simulink model "uz_FOC"  (R2021a)
settings: Solver=FixedStepDiscrete  StartTime=0.0  StopTime=50.0  FixedStep=0.00001  RelTol=1e-3  EnableMultiTasking=on
values from neighbouring files (symbols this model uses):
  d_d_TMS = 0.005    [uz_FOC_init.m]
  d_f_c = 100000    [uz_FOC_init.m]
  d_i_max = 15    [uz_FOC_init.m]
  d_i_min = -d_i_max    (= -15)    [uz_FOC_init.m]
  d_J_Coupling_M_E = 2e-6    (= 2e-06)    [uz_FOC_init.m]
  d_J_Coupling_M_Ms = 2e-20    [uz_FOC_init.m]
  d_J_Ms_L = d_J_Ms_M    (= 1.26363648e-05)    [uz_FOC_init.m]
  d_J_Ms_M = 0.5*0.5*((0.5*d_d_Ms)^4)*3.14*d_l_Ms*d_rho_Ms    (= 1.26363648e-05)    [uz_FOC_init.m]
  d_Ki_id = d_Kp_id/d_Tn_id    (= 125)    [uz_FOC_init.m]
  d_Ki_iq = d_Kp_iq/d_Tn_iq    (= 125)    [uz_FOC_init.m]
  d_Ki_n = d_Kp_n/d_Tn_n    (= 0.003888)    [uz_FOC_init.m]
  d_Kp_id = d_L_d / (4*20/d_f_c)    (= 0.25)    [uz_FOC_init.m]
  d_Kp_iq = d_L_q / (4*20/d_f_c)    (= 0.375)    [uz_FOC_init.m]
  d_Kp_n = 0.00864*0.045    (= 0.0003888)    [uz_FOC_init.m]
  d_L_d = 0.0002    [uz_FOC_init.m]
  d_L_q = 0.0003    [uz_FOC_init.m]
  d_p = 4    [uz_FOC_init.m]
  d_psi_pm = 0.0075    [uz_FOC_init.m]
  d_R_ph = d_R_ph_ph/2    (= 0.1)    [uz_FOC_init.m]
  d_y_max = 10    [uz_FOC_init.m]
  d_y_min = -d_y_max    (= -10)    [uz_FOC_init.m]
undefined symbols (not defined in the file or in its folder): i_d, i_q, para, u_d, u_q
libraries: fl_lib x44, nesl_utility x27, ee_lib x21, simulink x8, spsabctodq0Lib x2, spsTriangleGeneratorLib x1, eeTransforms x1
(part 3 of 3)

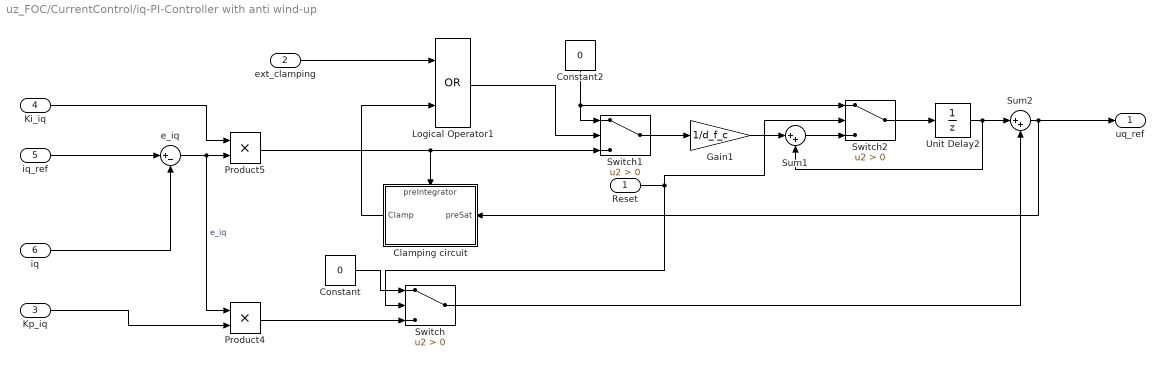
== system uz_FOC/CurrentControl/iq-PI-Controller with anti wind-up ==
  Reset : Inport
  ext_clamping : Inport  Port=2
  Kp_iq : Inport  Port=3
  Ki_iq : Inport  Port=4
  iq_ref : Inport  Port=5
  iq : Inport  Port=6
  Clamping circuit : Subsystem
      settings: PortSchema="{\"entries\":[{\"content\":{\"sides\":[{\"content\":{\"connectorIds\":[\"In1\"]},\"type\":\"ConnectorPlacement.EquallySpacedRectSide\",\"uuid\":\"9b5eb3d3-336d-4b55-a615-0420b1cf4a48\"},{\"content\":{\"connectorIds\":[\"Out1\"],\"side\":\"RIGHT\"},\"type\":\"ConnectorPlacement.EquallySpacedRectSide\",\"uuid\":\"a73559ab-79dd-4c84-b45a-6a43ba4812e9\"},{\"content\":{\"connectorIds\":[\"In2\"],\"side\":\"TOP\"},\"type\":\"ConnectorPlacement.EquallySpacedRectSide\",\"uuid\":\"82c30f31-c271-4a2b-89be-8686aa9e20f3\"}]},\"type\":\"ConnectorPlacement.EquallySpacedConnector\",\"uuid\":\"376d2fe4-39b3-495b-8d80-8756076e2730\"}],\"packageUris\":[\"http://schema.mathworks.com/mf0/Connector/R2020b\"],\"version\":\"1.0\"}"
  Constant : Constant  Value=0  SampleTime=1/d_f_c
  Constant2 : Constant  Value=0  SampleTime=1/d_f_c
  Gain1 : Gain  Gain=1/d_f_c
  Logical Operator1 : Logic  Operator=OR  AllPortsSameDT=off  OutDataTypeStr=boolean
  Product4 : Product
  Product5 : Product
  Sum1 : Sum  Inputs=|++  OutDataTypeStr=single
  Sum2 : Sum  Inputs=|++  OutDataTypeStr=single
  Switch : Switch  Criteria=u2 > Threshold
  Switch1 : Switch  Criteria=u2 > Threshold
  Switch2 : Switch  Criteria=u2 > Threshold
  Unit Delay2 : UnitDelay  SampleTime=-1  HasFrameUpgradeWarning=on
  e_iq : Sum  Inputs=|+-
  uq_ref : Outport
  wires:
  ext_clamping/1 -> Logical Operator1/1
  Kp_iq/1 -> Product4/2
  Ki_iq/1 -> Product5/1
  iq_ref/1 -> e_iq/1
  iq/1 -> e_iq/2
  e_iq/1 -> Product5/2, Product4/1  "e_iq"
  Unit Delay2/1 -> Sum2/1, Sum1/2
  Clamping circuit/1(Clamp) -> Logical Operator1/2
  Sum2/1 -> uq_ref/1, Clamping circuit/1(preSat)
  Switch/1 -> Sum2/2
  Constant/1 -> Switch/1
  Product4/1 -> Switch/3
  Switch2/1 -> Unit Delay2/1
  Gain1/1 -> Sum1/1
  Constant2/1 -> Switch2/1, Switch1/1
  Sum1/1 -> Switch2/3
  Product5/1 -> Switch1/3, Clamping circuit/2(preIntegrator)
  Switch1/1 -> Gain1/1
  Reset/1 -> Switch2/2, Switch/2
  Logical Operator1/1 -> Switch1/2

== system uz_FOC/CurrentControl/linear decouppling ==
  i_q : Inport
  i_d : Inport  Port=2
  omega_el : Inport  Port=3
  Gain : Gain  Gain=-d_L_q
  Gain4 : Gain  Gain=d_L_d
  Product : Product  SaturateOnIntegerOverflow=on
  Product1 : Product  SaturateOnIntegerOverflow=on
  Sum : Sum  Inputs=|++
  d_psi_pm : Constant  Value=d_psi_pm  OutDataTypeStr=Inherit: Inherit via back propagation  SampleTime=1/d_f_c
  u_d_vor : Outport  VectorParamsAs1DForOutWhenUnconnected=off
  u_q_vor : Outport  Port=2  VectorParamsAs1DForOutWhenUnconnected=off
  wires:
  i_q/1 -> Product/1
  Product1/1 -> u_q_vor/1
  Gain/1 -> Product/2
  Sum/1 -> Product1/1
  Product/1 -> u_d_vor/1
  omega_el/1 -> Gain/1, Product1/2
  Gain4/1 -> Sum/1
  d_psi_pm/1 -> Sum/2
  i_d/1 -> Gain4/1

== system uz_FOC/CurrentControl/nonlinear decouppling ==
  i_q : Inport
  i_d : Inport  Port=2
  omega_el : Inport  Port=3
  Gain12 : Gain  Gain=-1
  Product1 : Product
  Product8 : Product
  psi_d(u1=id,u2=iq) : Lookup_n-D  BreakpointsForDimension1=para.id_LUT  BreakpointsForDimension2=para.iq_LUT  Table=para.psi_q  InterpMethod=Cubic spline  ExtrapMethod=Clip  InternalRulePriority=Speed  RndMeth=Simplest  InputSameDT=on
      settings: InputPortMap=u0,u1
  psi_q(u1=id,u2=iq) : Lookup_n-D  BreakpointsForDimension1=para.id_LUT  BreakpointsForDimension2=para.iq_LUT  Table=para.psi_q  InterpMethod=Cubic spline  ExtrapMethod=Clip  InternalRulePriority=Speed  RndMeth=Simplest  InputSameDT=on
      settings: InputPortMap=u0,u1
  ud_vor : Outport  VectorParamsAs1DForOutWhenUnconnected=off
  uq_vor : Outport  Port=2  VectorParamsAs1DForOutWhenUnconnected=off
  wires:
  i_q/1 -> psi_q(u1=id,u2=iq)/2, psi_d(u1=id,u2=iq)/2
  i_d/1 -> psi_d(u1=id,u2=iq)/1, psi_q(u1=id,u2=iq)/1
  Product1/1 -> uq_vor/1
  Gain12/1 -> ud_vor/1
  Product8/1 -> Gain12/1
  psi_d(u1=id,u2=iq)/1 -> Product1/2
  omega_el/1 -> Product8/1, Product1/1
  psi_q(u1=id,u2=iq)/1 -> Product8/2

== system uz_FOC/Hardware/Coupling Encoder ==
  note: 1) Add Subsystem or Model blocks as valid variant choices.
      | 2) You cannot connect blocks at this level. At simulation, connectivity is automatically
      | determined, based on the active variant and port name matching.
  Inertia : Subsystem  VariantControl=(default)
  Spring Damper System : Subsystem  VariantControl=TMS1
  Input : PMIOPort  Side=Left
  output : PMIOPort  Port=2  Side=Right

== system uz_FOC/Hardware/Measurement Shaft ==
  note: 1) Add Subsystem or Model blocks as valid variant choices.
      | 2) You cannot connect blocks at this level. At simulation, connectivity is automatically
      | determined, based on the active variant and port name matching.
  Spring Damper System : Subsystem  VariantControl=TMS1
  default : Subsystem  VariantControl=(default)
  Input : PMIOPort  Side=Left
  output : PMIOPort  Port=2  Side=Right

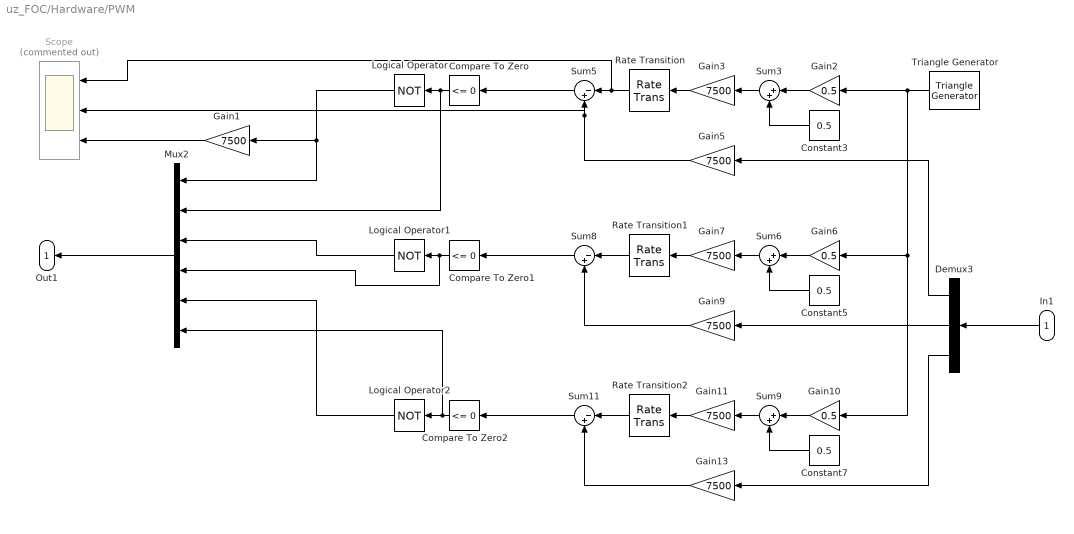
== system uz_FOC/Hardware/PWM ==
  In1 : Inport
  Compare To Zero : simulink/Logic and Bit Operations/Compare To Zero  relop=<=  OutDataTypeStr=boolean
  Compare To Zero1 : simulink/Logic and Bit Operations/Compare To Zero  relop=<=  OutDataTypeStr=boolean
  Compare To Zero2 : simulink/Logic and Bit Operations/Compare To Zero  relop=<=  OutDataTypeStr=boolean
  Constant3 : Constant  Value=0.5
  Constant5 : Constant  Value=0.5
  Constant7 : Constant  Value=0.5
  Demux3 : Demux  Outputs=3
  Gain{1,3,5,7,9,11,13} (7 alike) : Gain  Gain=7500  ParamDataTypeStr=single
  Gain10 : Gain  Gain=0.5
  Gain2 : Gain  Gain=0.5
  Gain6 : Gain  Gain=0.5
  Logical Operator : Logic  Operator=NOT  AllPortsSameDT=off  OutDataTypeStr=boolean
  Logical Operator1 : Logic  Operator=NOT  AllPortsSameDT=off  OutDataTypeStr=boolean
  Logical Operator2 : Logic  Operator=NOT  AllPortsSameDT=off  OutDataTypeStr=boolean
  Mux2 : Mux  Inputs=6
  Rate Transition : RateTransition  OutPortSampleTime=0.00001
  Rate Transition1 : RateTransition  OutPortSampleTime=0.00001
  Rate Transition2 : RateTransition  OutPortSampleTime=0.00001
  Scope : Scope  Commented=on  NumInputPorts=3
  Sum11 : Sum  Inputs=|-+
  Sum3 : Sum  Inputs=|++
  Sum5 : Sum  Inputs=|-+
  Sum6 : Sum  Inputs=|++
  Sum8 : Sum  Inputs=|-+
  Sum9 : Sum  Inputs=|++
  Triangle Generator : spsTriangleGeneratorLib/Triangle Generator  Freq=10000  Phase=0  Ts=0
  Out1 : Outport  VectorParamsAs1DForOutWhenUnconnected=off
  wires:
  Demux3/3 -> Gain13/1
  Logical Operator2/1 -> Mux2/5
  Logical Operator1/1 -> Mux2/3
  Mux2/1 -> Out1/1
  Compare To Zero2/1 -> Mux2/6, Logical Operator2/1
  Gain10/1 -> Sum9/1
  Sum8/1 -> Compare To Zero1/1
  Gain6/1 -> Sum6/1
  Sum9/1 -> Gain11/1
  Triangle Generator/1 -> Gain10/1, Gain6/1, Gain2/1
  Sum6/1 -> Gain7/1
  Demux3/2 -> Gain9/1
  Compare To Zero1/1 -> Mux2/4, Logical Operator1/1
  Constant5/1 -> Sum6/2
  Constant7/1 -> Sum9/2
  Sum11/1 -> Compare To Zero2/1
  Sum3/1 -> Gain3/1
  Constant3/1 -> Sum3/2
  Demux3/1 -> Gain5/1
  Sum5/1 -> Compare To Zero/1
  Gain2/1 -> Sum3/1
  In1/1 -> Demux3/1
  Gain3/1 -> Rate Transition/1
  Gain7/1 -> Rate Transition1/1
  Gain11/1 -> Rate Transition2/1
  Gain5/1 -> Scope/2, Sum5/2
  Gain9/1 -> Sum8/2
  Gain13/1 -> Sum11/2
  Rate Transition/1 -> Scope/1, Sum5/1
  Rate Transition1/1 -> Sum8/1
  Rate Transition2/1 -> Sum11/1
  Logical Operator/1 -> Gain1/1, Mux2/1
  Compare To Zero/1 -> Mux2/2, Logical Operator/1
  Gain1/1 -> Scope/3

== system uz_FOC/Hardware/Switch f. TMS ==
  note: 1) Add Subsystem or Model blocks as valid variant choices.
      | 2) You cannot connect blocks at this level. At simulation, connectivity is automatically
      | determined, based on the active variant and port name matching.
  closed : Subsystem  VariantControl=d_KupplZus==1
  open : Subsystem  VariantControl=d_KupplZus==0
  Input : PMIOPort  Side=Left
  output : PMIOPort  Port=2  Side=Right

== system uz_FOC/Hardware/coupling m. shaft ==
  note: 1) Add Subsystem or Model blocks as valid variant choices.
      | 2) You cannot connect blocks at this level. At simulation, connectivity is automatically
      | determined, based on the active variant and port name matching.
  Inertia : Subsystem  VariantControl=(default)
  Spring Damper System : Subsystem  VariantControl=TMS1
  Input : PMIOPort  Side=Left
  output : PMIOPort  Port=2  Side=Right

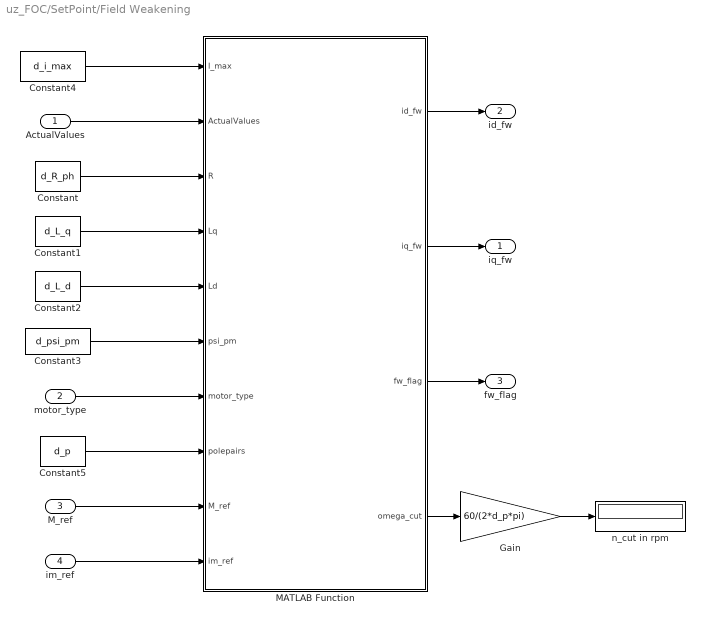
== system uz_FOC/SetPoint/Field Weakening ==
  ActualValues : Inport  OutDataTypeStr=single
  motor_type : Inport  Port=2  OutDataTypeStr=uint16
  M_ref : Inport  Port=3  OutDataTypeStr=single
  im_ref : Inport  Port=4  OutDataTypeStr=single
  Constant : Constant  Value=d_R_ph  OutDataTypeStr=single
  Constant1 : Constant  Value=d_L_q  OutDataTypeStr=single
  Constant2 : Constant  Value=d_L_d  OutDataTypeStr=single
  Constant3 : Constant  Value=d_psi_pm  OutDataTypeStr=single
  Constant4 : Constant  Value=d_i_max  OutDataTypeStr=single
  Constant5 : Constant  Value=d_p  OutDataTypeStr=single
  Gain : Gain  Gain=60/(2*d_p*pi)
  MATLAB Function : MATLAB Function  TreatAsAtomicUnit=on
  n_cut in rpm : Display
  iq_fw : Outport  OutDataTypeStr=single
  id_fw : Outport  Port=2  OutDataTypeStr=single
  fw_flag : Outport  Port=3  OutDataTypeStr=boolean
  wires:
  Constant4/1 -> MATLAB Function/1(I_max)
  ActualValues/1 -> MATLAB Function/2(ActualValues)
  Constant/1 -> MATLAB Function/3(R)
  Constant1/1 -> MATLAB Function/4(Lq)
  Constant2/1 -> MATLAB Function/5(Ld)
  Constant3/1 -> MATLAB Function/6(psi_pm)
  MATLAB Function/2(iq_fw) -> iq_fw/1
  MATLAB Function/1(id_fw) -> id_fw/1
  motor_type/1 -> MATLAB Function/7(motor_type)
  MATLAB Function/3(fw_flag) -> fw_flag/1
  M_ref/1 -> MATLAB Function/9(M_ref)
  im_ref/1 -> MATLAB Function/10(im_ref)
  Constant5/1 -> MATLAB Function/8(polepairs)
  MATLAB Function/4(omega_cut) -> Gain/1
  Gain/1 -> n_cut in rpm/1

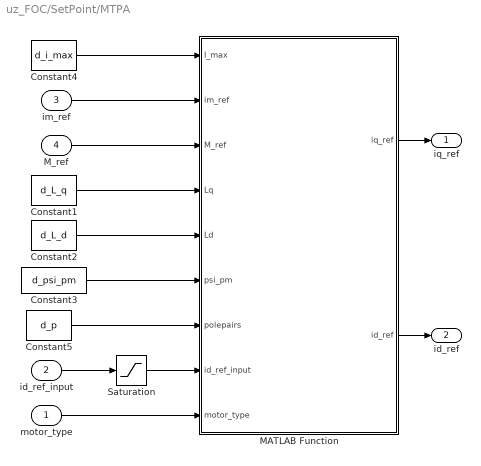
== system uz_FOC/SetPoint/MTPA ==
  motor_type : Inport  OutDataTypeStr=uint16
  id_ref_input : Inport  Port=2  OutDataTypeStr=single
  im_ref : Inport  Port=3  OutDataTypeStr=single
  M_ref : Inport  Port=4  OutDataTypeStr=single
  Constant1 : Constant  Value=d_L_q  OutDataTypeStr=single
  Constant2 : Constant  Value=d_L_d  OutDataTypeStr=single
  Constant3 : Constant  Value=d_psi_pm  OutDataTypeStr=single
  Constant4 : Constant  Value=d_i_max  OutDataTypeStr=single
  Constant5 : Constant  Value=d_p  OutDataTypeStr=single
  MATLAB Function : MATLAB Function  TreatAsAtomicUnit=on
  Saturation : Saturate  UpperLimit=d_i_max  LowerLimit=d_i_min
  iq_ref : Outport  OutDataTypeStr=single
  id_ref : Outport  Port=2  OutDataTypeStr=single
  wires:
  Constant4/1 -> MATLAB Function/1(I_max)
  Constant1/1 -> MATLAB Function/4(Lq)
  Constant2/1 -> MATLAB Function/5(Ld)
  Constant3/1 -> MATLAB Function/6(psi_pm)
  MATLAB Function/2(id_ref) -> id_ref/1
  MATLAB Function/1(iq_ref) -> iq_ref/1
  id_ref_input/1 -> Saturation/1
  Saturation/1 -> MATLAB Function/8(id_ref_input)
  im_ref/1 -> MATLAB Function/2(im_ref)
  motor_type/1 -> MATLAB Function/9(motor_type)
  Constant5/1 -> MATLAB Function/7(polepairs)
  M_ref/1 -> MATLAB Function/3(M_ref)

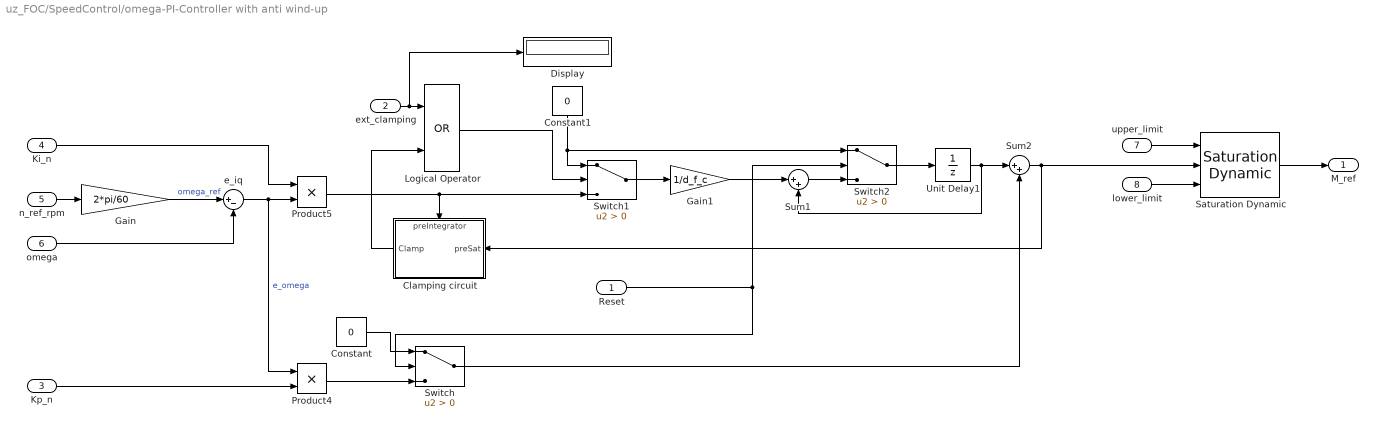
== system uz_FOC/SpeedControl/omega-PI-Controller with anti wind-up ==
  Reset : Inport
  ext_clamping : Inport  Port=2
  Kp_n : Inport  Port=3
  Ki_n : Inport  Port=4
  n_ref_rpm : Inport  Port=5
  omega : Inport  Port=6
  upper_limit : Inport  Port=7
  lower_limit : Inport  Port=8
  Clamping circuit : Subsystem
      settings: PortSchema="{\"entries\":[{\"content\":{\"sides\":[{\"content\":{\"connectorIds\":[\"In1\"]},\"type\":\"ConnectorPlacement.EquallySpacedRectSide\",\"uuid\":\"9b5eb3d3-336d-4b55-a615-0420b1cf4a48\"},{\"content\":{\"connectorIds\":[\"Out1\"],\"side\":\"RIGHT\"},\"type\":\"ConnectorPlacement.EquallySpacedRectSide\",\"uuid\":\"a73559ab-79dd-4c84-b45a-6a43ba4812e9\"},{\"content\":{\"connectorIds\":[\"In2\"],\"side\":\"TOP\"},\"type\":\"ConnectorPlacement.EquallySpacedRectSide\",\"uuid\":\"82c30f31-c271-4a2b-89be-8686aa9e20f3\"}]},\"type\":\"ConnectorPlacement.EquallySpacedConnector\",\"uuid\":\"376d2fe4-39b3-495b-8d80-8756076e2730\"}],\"packageUris\":[\"http://schema.mathworks.com/mf0/Connector/R2020b\"],\"version\":\"1.0\"}"
  Constant : Constant  Value=0  SampleTime=1/d_f_c
  Constant1 : Constant  Value=0  SampleTime=1/d_f_c
  Display : Display
  Gain : Gain  Gain=2*pi/60
  Gain1 : Gain  Gain=1/d_f_c
  Logical Operator : Logic  Operator=OR  AllPortsSameDT=off  OutDataTypeStr=boolean
  Product4 : Product
  Product5 : Product
  Saturation Dynamic : simulink/Discontinuities/Saturation Dynamic  OutMin=[]  OutMax=[]  OutDataTypeStr=Inherit: Same as second input  OutDataType=fixdt(1, 16)  OutScaling=2^-10  DoSatur=off
  Sum1 : Sum  Inputs=|++  OutDataTypeStr=single
  Sum2 : Sum  Inputs=|++  OutDataTypeStr=single
  Switch : Switch  Criteria=u2 > Threshold
  Switch1 : Switch  Criteria=u2 > Threshold
  Switch2 : Switch  Criteria=u2 > Threshold  OutDataTypeStr=single
  Unit Delay1 : UnitDelay  SampleTime=-1  HasFrameUpgradeWarning=on
  e_iq : Sum  Inputs=|+-  OutDataTypeStr=single
  M_ref : Outport
  wires:
  Kp_n/1 -> Product4/2
  Ki_n/1 -> Product5/1
  Gain/1 -> e_iq/1  "omega_ref"
  omega/1 -> e_iq/2
  e_iq/1 -> Product5/2, Product4/1  "e_omega"
  Switch/1 -> Sum2/2
  Unit Delay1/1 -> Sum2/1, Sum1/2
  Sum2/1 -> Clamping circuit/1(preSat), Saturation Dynamic/2
  ext_clamping/1 -> Display/1, Logical Operator/1
  Product5/1 -> Switch1/3, Clamping circuit/2(preIntegrator)
  Clamping circuit/1(Clamp) -> Logical Operator/2
  Constant/1 -> Switch/1
  Reset/1 -> Switch/2, Switch2/2
  Product4/1 -> Switch/3
  Constant1/1 -> Switch2/1, Switch1/1
  Logical Operator/1 -> Switch1/2
  n_ref_rpm/1 -> Gain/1
  Switch1/1 -> Gain1/1
  Gain1/1 -> Sum1/1
  Switch2/1 -> Unit Delay1/1
  Sum1/1 -> Switch2/3
  Saturation Dynamic/1 -> M_ref/1
  upper_limit/1 -> Saturation Dynamic/1
  lower_limit/1 -> Saturation Dynamic/3

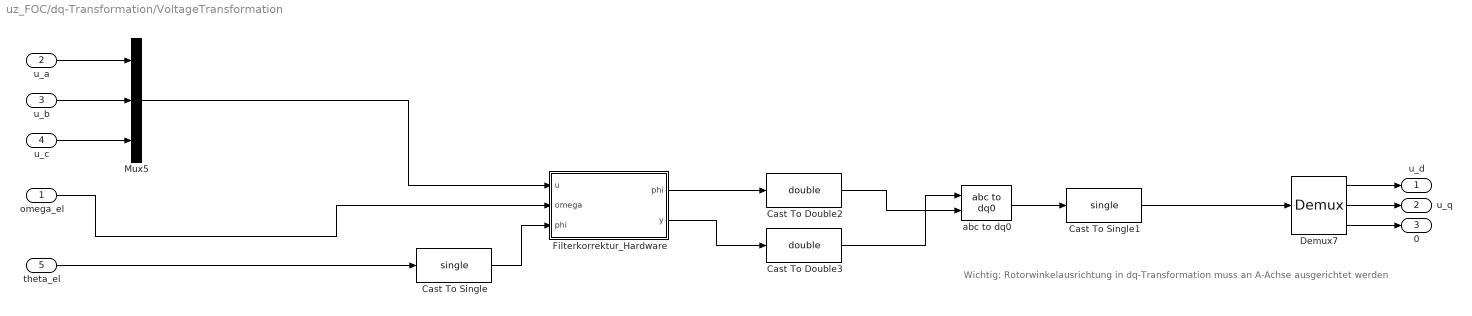
== system uz_FOC/dq-Transformation/VoltageTransformation ==
  note: Wichtig: Rotorwinkelausrichtung in dq-Transformation
      | muss an A-Achse ausgerichtet werden
  omega_el : Inport
  u_a : Inport  Port=2
  u_b : Inport  Port=3
  u_c : Inport  Port=4
  theta_el : Inport  Port=5
  Cast To Double2 : DataTypeConversion  OutDataTypeStr=double
  Cast To Double3 : DataTypeConversion  OutDataTypeStr=double
  Cast To Single : DataTypeConversion  OutDataTypeStr=single
  Cast To Single1 : DataTypeConversion  OutDataTypeStr=single
  Demux7 : Demux  Outputs=3
  Filterkorrektur_Hardware : MATLAB Function  TreatAsAtomicUnit=on
  Mux5 : Mux  Inputs=3
  abc to dq0 : spsabctodq0Lib/abc to dq0  Alignment=Aligned with phase A axis
  u_d : Outport  VectorParamsAs1DForOutWhenUnconnected=off
  u_q : Outport  Port=2  VectorParamsAs1DForOutWhenUnconnected=off
  0 : Outport  Port=3  VectorParamsAs1DForOutWhenUnconnected=off
  wires:
  Demux7/1 -> u_d/1
  Cast To Single/1 -> Filterkorrektur_Hardware/3("phi ")
  theta_el/1 -> Cast To Single/1
  Mux5/1 -> Filterkorrektur_Hardware/1(u)
  omega_el/1 -> Filterkorrektur_Hardware/2(omega)
  u_a/1 -> Mux5/1
  u_c/1 -> Mux5/3
  u_b/1 -> Mux5/2
  Demux7/3 -> 0/1
  Demux7/2 -> u_q/1
  Filterkorrektur_Hardware/1(phi) -> Cast To Double2/1
  Cast To Double2/1 -> abc to dq0/2
  Filterkorrektur_Hardware/2(y) -> Cast To Double3/1
  Cast To Double3/1 -> abc to dq0/1
  Cast To Single1/1 -> Demux7/1
  abc to dq0/1 -> Cast To Single1/1

== system uz_FOC/CurrentControl/id-PI-Controller with anti wind-up/Clamping circuit ==
  preSat : Inport  DisableCoverage=on  OutDataTypeStr=single
  preIntegrator : Inport  DisableCoverage=on  Port=2
  AND : Logic  DisableCoverage=on
  DataTypeConv1 : DataTypeConversion  DisableCoverage=on  OutDataTypeStr=int8  SaturateOnIntegerOverflow=on  RndMeth=Zero  LockScale=on
  DataTypeConv2 : DataTypeConversion  DisableCoverage=on  OutDataTypeStr=int8  SaturateOnIntegerOverflow=on  RndMeth=Zero  LockScale=on
  DeadZone : DeadZone  DisableCoverage=on  LowerValue=d_y_min  UpperValue=d_y_max  SaturateOnIntegerOverflow=on
  Equal : RelationalOperator  DisableCoverage=on  Operator===  RndMeth=Nearest  InputSameDT=on
  NotEqual : RelationalOperator  DisableCoverage=on  Operator=~=  RndMeth=Nearest  InputSameDT=on
  SignDeltaU : Signum  DisableCoverage=on
  SignPreIntegrator : Signum  DisableCoverage=on
  ZeroGain : Gain  DisableCoverage=on  Gain=0  ParamDataTypeStr=double  OutDataTypeStr=single  SaturateOnIntegerOverflow=on
  Clamp : Outport  DisableCoverage=on  VectorParamsAs1DForOutWhenUnconnected=off
  wires:
  preSat/1 -> ZeroGain/1, DeadZone/1
  preIntegrator/1 -> SignPreIntegrator/1
  ZeroGain/1 -> NotEqual/1
  DeadZone/1 -> NotEqual/2, SignDeltaU/1
  SignDeltaU/1 -> DataTypeConv1/1
  DataTypeConv1/1 -> Equal/1
  SignPreIntegrator/1 -> DataTypeConv2/1
  DataTypeConv2/1 -> Equal/2
  NotEqual/1 -> AND/1
  Equal/1 -> AND/2
  AND/1 -> Clamp/1

== system uz_FOC/CurrentControl/iq-PI-Controller with anti wind-up/Clamping circuit ==
  preSat : Inport  DisableCoverage=on  OutDataTypeStr=single
  preIntegrator : Inport  DisableCoverage=on  Port=2
  AND : Logic  DisableCoverage=on
  DataTypeConv1 : DataTypeConversion  DisableCoverage=on  OutDataTypeStr=int8  SaturateOnIntegerOverflow=on  RndMeth=Zero  LockScale=on
  DataTypeConv2 : DataTypeConversion  DisableCoverage=on  OutDataTypeStr=int8  SaturateOnIntegerOverflow=on  RndMeth=Zero  LockScale=on
  DeadZone : DeadZone  DisableCoverage=on  LowerValue=d_y_min  UpperValue=d_y_max  SaturateOnIntegerOverflow=on
  Equal : RelationalOperator  DisableCoverage=on  Operator===  RndMeth=Nearest  InputSameDT=on
  NotEqual : RelationalOperator  DisableCoverage=on  Operator=~=  RndMeth=Nearest  InputSameDT=on
  SignDeltaU : Signum  DisableCoverage=on
  SignPreIntegrator : Signum  DisableCoverage=on
  ZeroGain : Gain  DisableCoverage=on  Gain=0  ParamDataTypeStr=double  OutDataTypeStr=single  SaturateOnIntegerOverflow=on
  Clamp : Outport  DisableCoverage=on  VectorParamsAs1DForOutWhenUnconnected=off
  wires:
  preSat/1 -> ZeroGain/1, DeadZone/1
  preIntegrator/1 -> SignPreIntegrator/1
  ZeroGain/1 -> NotEqual/1
  DeadZone/1 -> NotEqual/2, SignDeltaU/1
  SignDeltaU/1 -> DataTypeConv1/1
  DataTypeConv1/1 -> Equal/1
  SignPreIntegrator/1 -> DataTypeConv2/1
  DataTypeConv2/1 -> Equal/2
  NotEqual/1 -> AND/1
  Equal/1 -> AND/2
  AND/1 -> Clamp/1

== system uz_FOC/Hardware/Coupling Encoder/Inertia ==
  Trägheitsmoment3 : fl_lib/Mechanical/Rotational Elements/Inertia  Commented=on  inertia=d_J_Coupling_M_E kg*m^2  num_ports=foundation.enum.numPorts2.one  w_specify=off  w_priority=High  w=0 rad/s  w_nominal_specify=off  w_nominal_unit=rad/s  w_nominal_value=1  t_specify=off  t_priority=None  t=0 N*m  t_nominal_specify=off  t_nominal_unit=N*m  t_nominal_value=1
      settings: AttributesFormatString=J in [%<inertia_unit>]
  Input : PMIOPort  Side=Left
  output : PMIOPort  Port=2  Side=Right
  connections:
  Input/RConn1 -- Trägheitsmoment3/LConn1 -- output/RConn1

== system uz_FOC/Hardware/Coupling Encoder/Spring Damper System ==
  Rotational Spring : fl_lib/Mechanical/Rotational Elements/Rotational Spring  spr_rate=d_c_Coupling_M_E N*m/rad  w_specify=off  w_priority=None  w=0 rad/s  w_nominal_specify=off  w_nominal_unit=rad/s  w_nominal_value=1  t_specify=off  t_priority=None  t=0 N*m  t_nominal_specify=off  t_nominal_unit=N*m  t_nominal_value=1  phi_specify=off  phi_priority=High  phi=0 rad  phi_nominal_specify=off  phi_nominal_unit=rad  phi_nominal_value=1
  Trägheitsmoment1 : fl_lib/Mechanical/Rotational Elements/Inertia  inertia=d_J_Coupling_M_E/2 kg*m^2  num_ports=foundation.enum.numPorts2.one  w_specify=off  w_priority=High  w=0 rad/s  w_nominal_specify=off  w_nominal_unit=rad/s  w_nominal_value=1  t_specify=off  t_priority=None  t=0 N*m  t_nominal_specify=off  t_nominal_unit=N*m  t_nominal_value=1
      settings: AttributesFormatString=J in [%<inertia_unit>]
  Trägheitsmoment3 : fl_lib/Mechanical/Rotational Elements/Inertia  inertia=d_J_Coupling_M_E/2 kg*m^2  num_ports=foundation.enum.numPorts2.one  w_specify=off  w_priority=High  w=0 rad/s  w_nominal_specify=off  w_nominal_unit=rad/s  w_nominal_value=1  t_specify=off  t_priority=None  t=0 N*m  t_nominal_specify=off  t_nominal_unit=N*m  t_nominal_value=1
      settings: AttributesFormatString=J in [%<inertia_unit>]
  dm : fl_lib/Mechanical/Rotational Elements/Rotational Damper  Commented=on  D=0 N*m/(rad/s)  w_specify=off  w_priority=None  w=0 rad/s  w_nominal_specify=off  w_nominal_unit=rad/s  w_nominal_value=1  t_specify=off  t_priority=None  t=0 N*m  t_nominal_specify=off  t_nominal_unit=N*m  t_nominal_value=1
  Input : PMIOPort  Side=Left
  output : PMIOPort  Port=2  Side=Right
  connections:
  Rotational Spring/LConn1 -- dm/LConn1 -- Input/RConn1 -- Trägheitsmoment3/LConn1
  Trägheitsmoment1/LConn1 -- Rotational Spring/RConn1 -- dm/RConn1 -- output/RConn1

== system uz_FOC/Hardware/Measurement Shaft/Spring Damper System ==
  Rotational Spring : fl_lib/Mechanical/Rotational Elements/Rotational Spring  spr_rate=d_c_Ms N*m/rad  w_specify=off  w_priority=None  w=0 rad/s  w_nominal_specify=off  w_nominal_unit=rad/s  w_nominal_value=1  t_specify=off  t_priority=None  t=0 N*m  t_nominal_specify=off  t_nominal_unit=N*m  t_nominal_value=1  phi_specify=off  phi_priority=High  phi=0 rad  phi_nominal_specify=off  phi_nominal_unit=rad  phi_nominal_value=1
  Trägheitsmoment1 : fl_lib/Mechanical/Rotational Elements/Inertia  inertia=d_J_Ms_L kg*m^2  num_ports=foundation.enum.numPorts2.one  w_specify=off  w_priority=High  w=0 rad/s  w_nominal_specify=off  w_nominal_unit=rad/s  w_nominal_value=1  t_specify=off  t_priority=None  t=0 N*m  t_nominal_specify=off  t_nominal_unit=N*m  t_nominal_value=1
      settings: AttributesFormatString=J in [%<inertia_unit>]
  Trägheitsmoment3 : fl_lib/Mechanical/Rotational Elements/Inertia  inertia=d_J_Ms_M kg*m^2  num_ports=foundation.enum.numPorts2.one  w_specify=off  w_priority=High  w=0 rad/s  w_nominal_specify=off  w_nominal_unit=rad/s  w_nominal_value=1  t_specify=off  t_priority=None  t=0 N*m  t_nominal_specify=off  t_nominal_unit=N*m  t_nominal_value=1
      settings: AttributesFormatString=J in [%<inertia_unit>]
  dm : fl_lib/Mechanical/Rotational Elements/Rotational Damper  D=d_d_TMS N*m/(rad/s)  w_specify=off  w_priority=None  w=0 rad/s  w_nominal_specify=off  w_nominal_unit=rad/s  w_nominal_value=1  t_specify=off  t_priority=None  t=0 N*m  t_nominal_specify=off  t_nominal_unit=N*m  t_nominal_value=1
  Input : PMIOPort  Side=Left
  output : PMIOPort  Port=2  Side=Right
  connections:
  Rotational Spring/LConn1 -- dm/LConn1 -- Trägheitsmoment3/LConn1 -- Input/RConn1
  Rotational Spring/RConn1 -- dm/RConn1 -- output/RConn1 -- Trägheitsmoment1/LConn1

== system uz_FOC/Hardware/Measurement Shaft/default ==
  Trägheitsmoment3 : fl_lib/Mechanical/Rotational Elements/Inertia  inertia=d_J_Ms_M+d_J_Ms_L kg*m^2  num_ports=foundation.enum.numPorts2.one  w_specify=off  w_priority=High  w=0 rad/s  w_nominal_specify=off  w_nominal_unit=rad/s  w_nominal_value=1  t_specify=off  t_priority=None  t=0 N*m  t_nominal_specify=off  t_nominal_unit=N*m  t_nominal_value=1
      settings: AttributesFormatString=J in [%<inertia_unit>]
  Input : PMIOPort  Side=Left
  output : PMIOPort  Port=2  Side=Right
  connections:
  Trägheitsmoment3/LConn1 -- output/RConn1 -- Input/RConn1

== system uz_FOC/Hardware/Switch f. TMS/closed ==
  Input : PMIOPort  Side=Left
  output : PMIOPort  Port=2  Side=Right
  connections:
  output/RConn1 -- Input/RConn1

== system uz_FOC/Hardware/Switch f. TMS/open ==
  Rotational Free End : fl_lib/Mechanical/Rotational Elements/Rotational Free End  w_specify=off  w_priority=None  w=0 rad/s  w_nominal_specify=off  w_nominal_unit=rad/s  w_nominal_value=1
      settings: SourceProductBaseCode=SS
  Rotational Free End1 : fl_lib/Mechanical/Rotational Elements/Rotational Free End  w_specify=off  w_priority=None  w=0 rad/s  w_nominal_specify=off  w_nominal_unit=rad/s  w_nominal_value=1
      settings: SourceProductBaseCode=SS
  Input : PMIOPort  Side=Left
  output : PMIOPort  Port=2  Side=Right
  connections:
  Rotational Free End1/LConn1 -- output/RConn1
  Input/RConn1 -- Rotational Free End/LConn1

== system uz_FOC/Hardware/coupling m. shaft/Inertia ==
  Trägheitsmoment3 : fl_lib/Mechanical/Rotational Elements/Inertia  Commented=on  inertia=d_J_Coupling_M_Ms kg*m^2  num_ports=foundation.enum.numPorts2.one  w_specify=off  w_priority=High  w=0 rad/s  w_nominal_specify=off  w_nominal_unit=rad/s  w_nominal_value=1  t_specify=off  t_priority=None  t=0 N*m  t_nominal_specify=off  t_nominal_unit=N*m  t_nominal_value=1
      settings: AttributesFormatString=J in [%<inertia_unit>]
  Input : PMIOPort  Side=Left
  output : PMIOPort  Port=2  Side=Right
  connections:
  Input/RConn1 -- Trägheitsmoment3/LConn1 -- output/RConn1

== system uz_FOC/Hardware/coupling m. shaft/Spring Damper System ==
  Rotational Spring : fl_lib/Mechanical/Rotational Elements/Rotational Spring  spr_rate=d_c_Coupling_M_Ms N*m/rad  w_specify=off  w_priority=None  w=0 rad/s  w_nominal_specify=off  w_nominal_unit=rad/s  w_nominal_value=1  t_specify=off  t_priority=None  t=0 N*m  t_nominal_specify=off  t_nominal_unit=N*m  t_nominal_value=1  phi_specify=off  phi_priority=High  phi=0 rad  phi_nominal_specify=off  phi_nominal_unit=rad  phi_nominal_value=1
  Trägheitsmoment1 : fl_lib/Mechanical/Rotational Elements/Inertia  inertia=d_J_Coupling_M_Ms/2 kg*m^2  num_ports=foundation.enum.numPorts2.one  w_specify=off  w_priority=High  w=0 rad/s  w_nominal_specify=off  w_nominal_unit=rad/s  w_nominal_value=1  t_specify=off  t_priority=None  t=0 N*m  t_nominal_specify=off  t_nominal_unit=N*m  t_nominal_value=1
      settings: AttributesFormatString=J in [%<inertia_unit>]
  Trägheitsmoment3 : fl_lib/Mechanical/Rotational Elements/Inertia  inertia=d_J_Coupling_M_Ms/2 kg*m^2  num_ports=foundation.enum.numPorts2.one  w_specify=off  w_priority=High  w=0 rad/s  w_nominal_specify=off  w_nominal_unit=rad/s  w_nominal_value=1  t_specify=off  t_priority=None  t=0 N*m  t_nominal_specify=off  t_nominal_unit=N*m  t_nominal_value=1
      settings: AttributesFormatString=J in [%<inertia_unit>]
  dm : fl_lib/Mechanical/Rotational Elements/Rotational Damper  Commented=on  D=0 N*m/(rad/s)  w_specify=off  w_priority=None  w=0 rad/s  w_nominal_specify=off  w_nominal_unit=rad/s  w_nominal_value=1  t_specify=off  t_priority=None  t=0 N*m  t_nominal_specify=off  t_nominal_unit=N*m  t_nominal_value=1
  Input : PMIOPort  Side=Left
  output : PMIOPort  Port=2  Side=Right
  connections:
  Rotational Spring/LConn1 -- dm/LConn1 -- Input/RConn1 -- Trägheitsmoment3/LConn1
  Trägheitsmoment1/LConn1 -- Rotational Spring/RConn1 -- dm/RConn1 -- output/RConn1

== system uz_FOC/SpeedControl/omega-PI-Controller with anti wind-up/Clamping circuit ==
  preSat : Inport  DisableCoverage=on  OutDataTypeStr=single
  preIntegrator : Inport  DisableCoverage=on  Port=2
  AND : Logic  DisableCoverage=on
  DataTypeConv1 : DataTypeConversion  DisableCoverage=on  OutDataTypeStr=int8  SaturateOnIntegerOverflow=on  RndMeth=Zero  LockScale=on
  DataTypeConv2 : DataTypeConversion  DisableCoverage=on  OutDataTypeStr=int8  SaturateOnIntegerOverflow=on  RndMeth=Zero  LockScale=on
  DeadZone : DeadZone  DisableCoverage=on  LowerValue=d_lower_limit  UpperValue=d_upper_limit  SaturateOnIntegerOverflow=on
  Equal : RelationalOperator  DisableCoverage=on  Operator===  RndMeth=Nearest  InputSameDT=on
  NotEqual : RelationalOperator  DisableCoverage=on  Operator=~=  RndMeth=Nearest  InputSameDT=on
  SignDeltaU : Signum  DisableCoverage=on
  SignPreIntegrator : Signum  DisableCoverage=on
  ZeroGain : Gain  DisableCoverage=on  Gain=0  ParamDataTypeStr=double  OutDataTypeStr=single  SaturateOnIntegerOverflow=on
  Clamp : Outport  DisableCoverage=on  VectorParamsAs1DForOutWhenUnconnected=off
  wires:
  preSat/1 -> ZeroGain/1, DeadZone/1
  preIntegrator/1 -> SignPreIntegrator/1
  ZeroGain/1 -> NotEqual/1
  DeadZone/1 -> NotEqual/2, SignDeltaU/1
  SignDeltaU/1 -> DataTypeConv1/1
  DataTypeConv1/1 -> Equal/1
  SignPreIntegrator/1 -> DataTypeConv2/1
  DataTypeConv2/1 -> Equal/2
  NotEqual/1 -> AND/1
  Equal/1 -> AND/2
  AND/1 -> Clamp/1

== matlab function uz_FOC/dq-Transformation/VoltageTransformation/Filterkorrektur_Hardware ==
  data: phi output; u input; y output; omega input; phi input

function [phi,y]= fcn(u,omega, phi)

R=95300;%ohm
RL=8200;%ohm
C=0.000000047;%Farrad
T=(RL*R*C)/(R+RL);

 w=omega;
%Filter zur Kompensation des Phasenversatz der Spannungen
 for i=single(1):single(3)
     %Rückgängigkmachen der ADC Umrechung und umkehren der Filterfunktion
u(i)=u(i)*(1/((R+RL)/RL))*(    ((R+RL)/RL)^2 + (w*R*C)^2          )^0.5;
 end
 

phi=(phi)- atan(  w*T   );%atan(  w*T   );%*(1.08);


y = u;

== matlab function uz_FOC/SetPoint/MTPA/MATLAB Function ==
  data: I_max input single; im_ref input; M_ref input; iq_ref output single; Lq input single; Ld input single; psi_pm input single; polepairs input; id_ref output; id_ref_input input; motor_type input
function [iq_ref, id_ref]= MTPA(I_max, im_ref, M_ref, Lq, Ld, psi_pm, polepairs, id_ref_input, motor_type)
if (M_ref ~= 0)
    
    if(motor_type==0)
        iq_ref = im_ref;
        id_temp = single(0);
    elseif(motor_type==1)
        %Approximation with newton-raphson algorithm
        iq_newton=im_ref;
        d=(2*M_ref*psi_pm)/(3*(Ld-Lq)^2*polepairs);
        e=((2*M_ref)^2)/(9*(Ld-Lq)^2*polepairs^2);

        for i=1:15
            iq_newton = iq_newton - (iq_newton^4 + d*iq_newton - e) / (4*iq_newton^3 + d);
        end
        if(iq_newton > 0)
            iq_ref = min(iq_newton, I_max);
        else
            iq_ref = max(iq_newton, -I_max);
        end
        if (Ld < Lq)
            id_temp = (-psi_pm / (2*(Ld - Lq))) - sqrt((psi_pm^2 / (4*(Ld - Lq)^2))+iq_ref^2 );
            id_temp = max(id_temp, -sqrt(I_max^2 - iq_ref^2));
        else
            id_temp = (-psi_pm / (2*(Ld - Lq))) + sqrt((psi_pm^2 / (4*(Ld - Lq)^2))+iq_ref^2 );
            id_temp = min(id_temp, sqrt(I_max^2 - iq_ref^2));
        end
    else
        id_temp = single(0);
        iq_ref = single(0);
    end

    id_ref = id_temp + id_ref_input;
    if(id_ref >0)
        id_ref = min(id_ref, sqrt(I_max^2 - iq_ref^2));
    else
        id_ref = max(id_ref, -sqrt(I_max^2 - iq_ref^2));
    end
else
    id_ref = single(0);
    iq_ref = single(0);
end

== matlab function uz_FOC/Space vector limitation ==
  data: VoltageReference input Bus: VoltageReference; ActualValues input; limit_on output boolean; Fehler output; Fall output; VoltageReference output
% Algorithm for voltage space vector limitation
% 
% Quelle:    Vector Control of Three-Phase AC Machines, S. 183
% Autoren:   Nguyen Phung Quang, Jörg-Andreas Dittrich
%            Springer, 2015,Second Edition


function [limit_on, Fehler, Fall,VoltageReference] = fcn(VoltageReference, ActualValues)
%#codegen

% maximale Amplitude des Raumzeigers bzw. der Leiterspannung
   % ohne Addition einer 3ten Harmonischen   U^_LN = U_ZK/2;
   %U_RZ_max = U_ZK*0.5;
   %bei Offsetaddition der 3te Harmonischen  U^_LN = U_ZK/sqrt(3);
   U_RZ_max =ActualValues.U_zk/sqrt(3);

% Betrag des Raumzeigers aus U_d und U_q
U_RZ_betrag = sqrt(VoltageReference.u_d_ref^2 + VoltageReference.u_q_ref^2);

% Ist eine Begrenzung notwendig?
if ( U_RZ_betrag > U_RZ_max)   
    limit_on = boolean(1);   % Begrenzung notwendig -> motorischer oder generatorischer Betrieb?
   
    if ((sign(ActualValues.omega_el)==sign(ActualValues.i_q)) ) % Motorbetrieb      
        Fehler = 0;
        if ( (abs(VoltageReference.u_d_ref) > 0.95*U_RZ_max) )
        %true
        U_d_limit = sign(VoltageReference.u_d_ref)*0.95*U_RZ_max;
        U_q_limit = sign(VoltageReference.u_q_ref)*sqrt(U_RZ_max^2-U_d_limit^2);
        Fall = 2;
        else
        %false
        U_d_limit = VoltageReference.u_d_ref;
        U_q_limit = sign(VoltageReference.u_q_ref)*sqrt(U_RZ_max^2-U_d_limit^2);
        Fall = 1;
        end    
    
    
    elseif ((sign(ActualValues.omega_el)~=sign(ActualValues.i_q)) ) % Generatorbetrieb   
        Fehler = 0;
        if ( abs(VoltageReference.u_q_ref) > 0.95*U_RZ_max )
        %true
        U_q_limit = sign(VoltageReference.u_q_ref)*0.95*U_RZ_max;
        U_d_limit = sign(VoltageReference.u_d_ref)*sqrt(U_RZ_max^2-U_q_limit^2);
        %U_d_limit = U_d;
        Fall = 4;       
        else 
        % false
        U_q_limit = VoltageReference.u_q_ref;
        U_d_limit = sign(VoltageReference.u_d_ref)*sqrt(U_RZ_max^2-U_q_limit^2);
        Fall = 3;
        end
        
    else % Weder motorischer noch generatorischer Betrieb => Fehler 
    U_d_limit = VoltageReference.u_d_ref;
    U_q_limit = VoltageReference.u_q_ref;
    Fehler = 1;
    Fall = 5;
    end
    
else
% keine Begrenzung notwendig
    U_d_limit = VoltageReference.u_d_ref;
    U_q_limit = VoltageReference.u_q_ref;
    limit_on = boolean(0);
    Fehler = 0;
    Fall = 0;
end
VoltageReference.u_d_ref = U_d_limit;
VoltageReference.u_q_ref = U_q_limit;
end

== matlab function uz_FOC/Hardware/12bit ADC ==
  data: u input; y output
function y = fcn(u)
%#codegen

y = u*2048/5;

== matlab function uz_FOC/Hardware/12bit ADC1 ==
  data: u input; y output
function y = fcn(u)
%#codegen

y = u*2048/5;

== matlab function uz_FOC/Hardware/12bit ADC2 ==
  data: u input; y output
function y = fcn(u)
%#codegen

y = u*2048/5;

== matlab function uz_FOC/SetPoint/Field Weakening/MATLAB Function ==
  data: I_max input single; id_fw output single; ActualValues input Bus: ActualValues; R input single; Lq input single; Ld input single; psi_pm input single; iq_fw output; motor_type input; fw_flag output; polepairs input; M_ref input single; im_ref input single; omega_cut output
function [id_fw, iq_fw, fw_flag, omega_cut]= field_weakening(I_max, ActualValues, R, Lq, Ld, psi_pm, motor_type, polepairs, M_ref, im_ref)

fw_flag = boolean(0);
%Maximum voltage vector
u_max_dq = single(ActualValues.U_zk/sqrt(single(3)) - R*I_max)*0.95;
I1 = sqrt(ActualValues.i_d^2 + ActualValues.i_q^2);
%Calculation of n_cut
a = single((I1^2 * Lq^2) + psi_pm^2);
b = single(2*R*psi_pm*abs(I1));
c = single((I1^2 * R^2)-u_max_dq^2);
omega_cut = single((-b + sqrt(b^2 - 4*a*c))/(2*a));

if(M_ref ~=0)
    %Check if w_cut is valid
    if omega_cut > 0 && isreal(single(omega_cut))  
        %Calcultation of Id_ref
        if abs(ActualValues.omega_el) > omega_cut
            fw_flag = boolean(1);
            if(motor_type == 0)
                id_fw = single(psi_pm/Ld * (omega_cut/abs(ActualValues.omega_el) -1));
                id_fw = max(id_fw, -I_max);
                if(ActualValues.omega_el >0)
                    iq_fw = min(im_ref, sqrt(I_max^2 - id_fw^2));
                else
                    iq_fw = max(im_ref, -sqrt(I_max^2 - id_fw^2));
                end
            elseif(motor_type == 1)
                %Approximation with newton-raphson algorithm
                if(ActualValues.omega_el > 0)
                    iq_fw = I_max /2;
                else
                    iq_fw = -I_max /2;
                end
                c = (psi_pm^2*Lq^2 - (Ld-Lq)^2 * u_max_dq^2 / ActualValues.omega_el^2) / (Lq^2*(Ld-Lq)^2);
                d=(-4*M_ref*Ld*Lq*psi_pm)/(3*(Ld-Lq)^2*polepairs*Lq^2);
                e=((2*M_ref*Ld)^2)/(9*(Ld-Lq)^2*polepairs^2*Lq^2);

                for i=1:15
                    iq_fw = iq_fw - (iq_fw^4 + c*iq_fw^2 + d*iq_fw + e) / (4*iq_fw^3 + 2*c*iq_fw + d);
                end
                if(iq_fw <0)           
                    iq_fw = max(iq_fw, -I_max);
                else          
                    iq_fw = min(iq_fw, I_max);
                end     
                id_fw = -(psi_pm/Ld) + 1/Ld * sqrt((u_max_dq/ActualValues.omega_el)^2 - (Lq*iq_fw)^2);
            else
                id_fw = single(0);
                iq_fw = single(0.0);
            end
            id_fw = max(id_fw, -sqrt(I_max^2 - iq_fw^2));
            if id_fw > 0
                id_fw = single(0.0);
            end
        else
            id_fw = single(0.0);
            iq_fw = single(0.0);
        end
    else
        id_fw = single(0.0);
        iq_fw = single(0.0);
    end

else
    id_fw = single(0);
    iq_fw = single(0);
end

== matlab function uz_FOC/Space Vector Modulation/MATLAB Function ==
  data: u_alpha input; CMP_U output; u_beta input; V_DC input; CMP_V output; CPM_W output
function [CMP_U, CMP_V, CPM_W] = fcn(u_alpha, u_beta, V_DC)

CMP_U=single(0);
CMP_V=single(0);
CPM_W=single(0);
a=single(0);
b=single(0);
c=single(0);

 %%__%%__%%__%%__%%__%%__%%__%%__%%__%%__%%__%%__%%__%%__%%__%%__%%__%%__%%_
    %%Space vecotr modulation%%
    %%Eingänge:
    %V_DC       -- DC-link voltage
    %u_alpha    -- alpha component of the reference space vector
    %u_beta     -- beta component of the reference space vector
    %%Ausgänge:
    %CMP_U        -- Comparsion value U
    %CMP_V        -- Comparsion value V
    %CMP_W        -- Comparsion value W
    
    
    %Calculation of a,b,c from Quang Dittrich S24
    
    a = (abs(u_alpha) + (1/sqrt(3))*abs(u_beta))/(2/3*V_DC);
    b = (abs(u_alpha) - (1/sqrt(3))*abs(u_beta))/(2/3*V_DC);
    c = ((2/sqrt(3))*abs(u_beta))/(2/3*V_DC);
    
    
    %sector and quadrants from Quang Dittrich S32
    if(u_beta < 0)
        if (u_alpha <0)
            quadrant=3;
            if(b < 0)
                sector = 5;
            else
                sector = 4;
            end
        else
            quadrant=4;
            if(b < 0)
                sector = 5;
            else
                sector = 6;
            end
        end
        
    else
        if (u_alpha <0)
            quadrant=2;
            if(b < 0)
                sector = 2;
            else
                sector = 3;
            end
        else
            quadrant=1;
            if(b < 0)
                sector = 2;
            else
                sector = 1;
            end
        end
    end

    %%modulation for phases U,V,W
    
    if (sector == 1)
        CMP_U = 0.5*(1 + b + c);
        CMP_V = 0.5*(1 - b + c);
        CPM_W = 0.5*(1 - b - c);
    end
    
    
    if ((sector == 2) && (quadrant == 1))        
        CMP_U = 0.5*(1 + a + b);
        CMP_V = 0.5*(1 + a - b);
        CPM_W = 0.5*(1 - a + b);
    end
    
    
    if ((sector == 2) && (quadrant == 2))
        CMP_U = 0.5*(1 - a - b);
        CMP_V = 0.5*(1 + a - b);
        CPM_W = 0.5*(1 - a + b);
    end
    
    
    if (sector == 3)
        CMP_U = 0.5*(1 - b - c);
        CMP_V = 0.5*(1 + b + c);
        CPM_W = 0.5*(1 + b - c);
    end
    
    if (sector == 4)
        CMP_U = 0.5*(1 - b - c);
        CMP_V = 0.5*(1 + b - c);
        CPM_W = 0.5*(1 + b + c);
    end
    
    
    if ((sector == 5) && (quadrant == 3))
        CMP_U = 0.5*(1 - a - b);
        CMP_V = 0.5*(1 - a + b);
        CPM_W = 0.5*(1 + a - b);
    end
    
    
    if ((sector == 5) && (quadrant == 4))
        CMP_U = 0.5*(1 + b + a);
        CMP_V = 0.5*(1 + b - a);
        CPM_W = 0.5*(1 - b + a);
    end
    
    
    if (sector == 6)
        CMP_U = 0.5*(1 + b + c);
        CMP_V = 0.5*(1 - b - c);
        CPM_W = 0.5*(1 - b + c);
    end

    
    %%Begrenzung
    if (CMP_U > 1)
        CMP_U = single(1);
    end
    if (CMP_U < 0)
        CMP_U = single(0);
    end
    
    if (CMP_V > 1)
        CMP_V = single(1);
    end
    if (CMP_V < 0)
        CMP_V = single(0);
    end
    
    if (CPM_W > 1)
        CPM_W = single(1);
    end
    if (CPM_W < 0)
        CPM_W = single(0);
    end
